simulink model "PTC_MBDS_StringToNumber_Sample"  (R2013a)
settings: Solver=FixedStepDiscrete  SolverMode=SingleTasking  StartTime=0.0  StopTime=100  FixedStep=0.02  RelTol=1e-3
libraries: PTC_MBDS_LIB x13, simulink_extras x1
CloseFcn:
  | rtwprivate ssgencode ModelCloseRequest MOD_Function6
Description:
  | Model of an MBDS Application
settings Model: CovPath=/Model  CovMetricSettings=dcmtrwa  CovHTMLOptions=-aTS=1 -bRG=1 -bTC=0 -hTR=0 -nFC=0 -scm=1 -bcm=1  covSaveCumulativeToWorkspaceVar=off  CovSaveSingleToWorkspaceVar=off  Creator=uid60719  LastModifiedBy=sundeep.tuteja
settings DataIOCC: LimitDataPoints=off  MaxDataPoints=100  SignalLoggingSaveFormat=ModelDataLogs  SaveOutput=off  SignalLogging=off  SaveTime=off
settings OptimizationCC: InlineParams=on  InlineInvariantSignals=on  ExpressionDepthLimit=2147483647  StateBitsets=on  DataBitsets=on  EfficientFloat2IntCast=on
settings DebuggingCC: ConsistencyChecking=error  SignalInfNanChecking=error  AlgebraicLoopMsg=error  ArtificialAlgebraicLoopMsg=error  SaveWithParameterizedLinksMsg=none  BlockPriorityViolationMsg=error  MinStepSizeMsg=error  SolverPrmCheckMsg=error  InheritedTsInSrcMsg=none  DiscreteInheritContinuousMsg=error  MultiTaskCondExecSysMsg=none  SingleTaskRateTransMsg=warning  TasksWithSamePriorityMsg=error  SigSpecEnsureSampleTimeMsg=error  CheckMatrixSingularityMsg=error  ParameterUnderflowMsg=error  UnnecessaryDatatypeConvMsg=warning  VectorMatrixConversionMsg=error  FcnCallInpInsideContextMsg=UseLocalSettings  SignalLabelMismatchMsg=warning  SFcnCompatibilityMsg=warning  UniqueDataStoreMsg=error  BusObjectLabelMismatch=error  RootOutportRequireBusObject=error  ModelReferenceIOMsg=warning  ModelReferenceVersionMismatchMessage=warning  ModelReferenceIOMismatchMessage=warning  ModelReferenceCSMismatchMessage=warning  UnknownTsInhSupMsg=error
settings HardwareCC: ProdIntDivRoundTo=Zero  ProdEndianess=BigEndian  ProdHWDeviceType=Specified  TargetHWDeviceType=32-bit Generic  ProdEqTarget=off
settings RTWCC: GenerateReport=on  ProcessScript=grt_make_rtw_hook  CustomInclude=dir c:\projects\siemensVDO\SV_MBDS\PLCLibrary\PLC\SVDO_Include\  LaunchReport=on  IncludeERTFirstTime=on
settings GRTTargetCC: CombineOutputUpdateFcns=off  GRTInterface=on

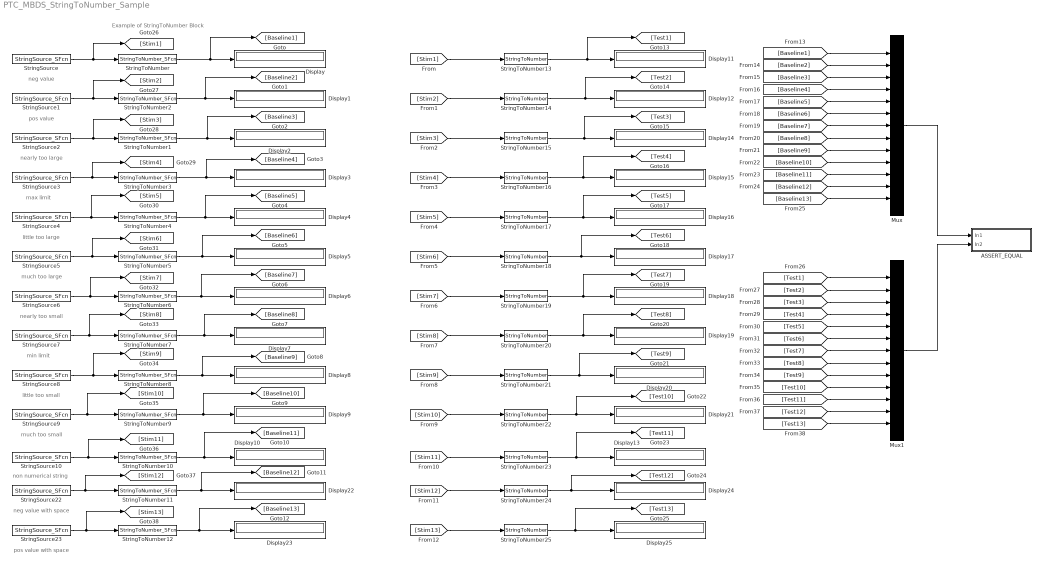
== system PTC_MBDS_StringToNumber_Sample ==
  note: neg value
  note: pos value
  note: nearly too large
  note: max limit
  note: little too large
  note: much too large
  note: nearly too small
  note: min limit
  note: little too small
  note: much too small
  note: non numerical string
  note: Example of StringToNumber Block
  note: neg value with space
  note: pos value with space
  ASSERT_EQUAL : Subsystem
  Display{,1..25} (26 alike) : Display
      settings: Format=decimal (Stored Integer)
  Mux : Mux  Inputs=13
  Mux1 : Mux  Inputs=13
  StringSource : S-Function  InitFcn=|  FunctionName=StringSource_SFcn  Parameters=uint8(String), uint16(MaxStringLength)  EnableBusSupport=off  mask(StringSource){MBDS_LibraryBlock=on, InputValue=-12345, MBDS_BlockVersion=05.20}
      | if(exist('MBDS_BlockCallback', 'file'))
      |    MBDS_BlockCallback('Update', gcb);
      | end
      mask prompts: MBDS_LibraryBlock "MBDS Library Block"; InputValue "Constant value:"; MBDS_BlockVersion "Block version:"
      mask help: This block outputs an uint8 array based on the ASCII codes of the string specified by the user.
      mask init:
      | MBDS_BlockCallback('Copy', gcb);
      | MaxStringLength = 1 + GetStringLen();
      | DispString = 'Error';
      | String = InputValue;
      | % Skip if string specifies a numeric expression or starts with '
      | if(isempty(str2num(String)) && String(1) ~= '''')
      |    try
      |       % Try to evaluate project constant 
      |       String = evalin('base', String);
      |    end   
      | end
      | if ~ischar(String) || size(String, 1) > 1
      | 	error('String must be a [1xn] array of type ''char'' with at least one character')
      | else
      |    % Limit to max. string length
      |    String = String(1:min(MaxStringLength, length(String)));
      | 	DispString = InputValue;
      | end
      mask Help: eval(['open([workdir(''Library_Dir:''),''\Blockset\Help\'',get_param(gcb,''MaskType''),''.html''])'])
      mask Display: text(0.05,0.5,DispString,'horizontalAlignment','left')
  StringSource1 : S-Function  InitFcn=|  FunctionName=StringSource_SFcn  Parameters=uint8(String), uint16(MaxStringLength)  EnableBusSupport=off  mask(StringSource){MBDS_LibraryBlock=on, InputValue=12345, MBDS_BlockVersion=05.20}
      | if(exist('MBDS_BlockCallback', 'file'))
      |    MBDS_BlockCallback('Update', gcb);
      | end
      mask prompts: MBDS_LibraryBlock "MBDS Library Block"; InputValue "Constant value:"; MBDS_BlockVersion "Block version:"
      mask help: This block outputs an uint8 array based on the ASCII codes of the string specified by the user.
      mask init: same as PTC_MBDS_StringToNumber_Sample/StringSource
      mask Help: eval(['open([workdir(''Library_Dir:''),''\Blockset\Help\'',get_param(gcb,''MaskType''),''.html''])'])
      mask Display: text(0.05,0.5,DispString,'horizontalAlignment','left')
  StringSource10 : S-Function  InitFcn=|  FunctionName=StringSource_SFcn  Parameters=uint8(String), uint16(MaxStringLength)  EnableBusSupport=off  mask(StringSource){MBDS_LibraryBlock=on, InputValue=1a23, MBDS_BlockVersion=05.20}
      | if(exist('MBDS_BlockCallback', 'file'))
      |    MBDS_BlockCallback('Update', gcb);
      | end
      mask prompts: MBDS_LibraryBlock "MBDS Library Block"; InputValue "Constant value:"; MBDS_BlockVersion "Block version:"
      mask help: This block outputs an uint8 array based on the ASCII codes of the string specified by the user.
      mask init: same as PTC_MBDS_StringToNumber_Sample/StringSource
      mask Help: eval(['open([workdir(''Library_Dir:''),''\Blockset\Help\'',get_param(gcb,''MaskType''),''.html''])'])
      mask Display: text(0.05,0.5,DispString,'horizontalAlignment','left')
  StringSource2 : S-Function  InitFcn=|  FunctionName=StringSource_SFcn  Parameters=uint8(String), uint16(MaxStringLength)  EnableBusSupport=off  mask(StringSource){MBDS_LibraryBlock=on, InputValue=2147483645, MBDS_BlockVersion=05.20}
      | if(exist('MBDS_BlockCallback', 'file'))
      |    MBDS_BlockCallback('Update', gcb);
      | end
      mask prompts: MBDS_LibraryBlock "MBDS Library Block"; InputValue "Constant value:"; MBDS_BlockVersion "Block version:"
      mask help: This block outputs an uint8 array based on the ASCII codes of the string specified by the user.
      mask init: same as PTC_MBDS_StringToNumber_Sample/StringSource
      mask Help: eval(['open([workdir(''Library_Dir:''),''\Blockset\Help\'',get_param(gcb,''MaskType''),''.html''])'])
      mask Display: text(0.05,0.5,DispString,'horizontalAlignment','left')
  StringSource22 : S-Function  InitFcn=|  FunctionName=StringSource_SFcn  Parameters=uint8(String), uint16(MaxStringLength)  EnableBusSupport=off  mask(StringSource){MBDS_LibraryBlock=on, InputValue=-12345, MBDS_BlockVersion=05.20}
      | if(exist('MBDS_BlockCallback', 'file'))
      |    MBDS_BlockCallback('Update', gcb);
      | end
      mask prompts: MBDS_LibraryBlock "MBDS Library Block"; InputValue "Constant value:"; MBDS_BlockVersion "Block version:"
      mask help: This block outputs an uint8 array based on the ASCII codes of the string specified by the user.
      mask init: same as PTC_MBDS_StringToNumber_Sample/StringSource
      mask Help: eval(['open([workdir(''Library_Dir:''),''\Blockset\Help\'',get_param(gcb,''MaskType''),''.html''])'])
      mask Display: text(0.05,0.5,DispString,'horizontalAlignment','left')
  StringSource23 : S-Function  InitFcn=|  FunctionName=StringSource_SFcn  Parameters=uint8(String), uint16(MaxStringLength)  EnableBusSupport=off  mask(StringSource){MBDS_LibraryBlock=on, InputValue=12345, MBDS_BlockVersion=05.20}
      | if(exist('MBDS_BlockCallback', 'file'))
      |    MBDS_BlockCallback('Update', gcb);
      | end
      mask prompts: MBDS_LibraryBlock "MBDS Library Block"; InputValue "Constant value:"; MBDS_BlockVersion "Block version:"
      mask help: This block outputs an uint8 array based on the ASCII codes of the string specified by the user.
      mask init: same as PTC_MBDS_StringToNumber_Sample/StringSource
      mask Help: eval(['open([workdir(''Library_Dir:''),''\Blockset\Help\'',get_param(gcb,''MaskType''),''.html''])'])
      mask Display: text(0.05,0.5,DispString,'horizontalAlignment','left')
  StringSource3 : S-Function  InitFcn=|  FunctionName=StringSource_SFcn  Parameters=uint8(String), uint16(MaxStringLength)  EnableBusSupport=off  mask(StringSource){MBDS_LibraryBlock=on, InputValue=2147483647, MBDS_BlockVersion=05.20}
      | if(exist('MBDS_BlockCallback', 'file'))
      |    MBDS_BlockCallback('Update', gcb);
      | end
      mask prompts: MBDS_LibraryBlock "MBDS Library Block"; InputValue "Constant value:"; MBDS_BlockVersion "Block version:"
      mask help: This block outputs an uint8 array based on the ASCII codes of the string specified by the user.
      mask init: same as PTC_MBDS_StringToNumber_Sample/StringSource
      mask Help: eval(['open([workdir(''Library_Dir:''),''\Blockset\Help\'',get_param(gcb,''MaskType''),''.html''])'])
      mask Display: text(0.05,0.5,DispString,'horizontalAlignment','left')
  StringSource4 : S-Function  InitFcn=|  FunctionName=StringSource_SFcn  Parameters=uint8(String), uint16(MaxStringLength)  EnableBusSupport=off  mask(StringSource){MBDS_LibraryBlock=on, InputValue=2147483648, MBDS_BlockVersion=05.20}
      | if(exist('MBDS_BlockCallback', 'file'))
      |    MBDS_BlockCallback('Update', gcb);
      | end
      mask prompts: MBDS_LibraryBlock "MBDS Library Block"; InputValue "Constant value:"; MBDS_BlockVersion "Block version:"
      mask help: This block outputs an uint8 array based on the ASCII codes of the string specified by the user.
      mask init: same as PTC_MBDS_StringToNumber_Sample/StringSource
      mask Help: eval(['open([workdir(''Library_Dir:''),''\Blockset\Help\'',get_param(gcb,''MaskType''),''.html''])'])
      mask Display: text(0.05,0.5,DispString,'horizontalAlignment','left')
  StringSource5 : S-Function  InitFcn=|  FunctionName=StringSource_SFcn  Parameters=uint8(String), uint16(MaxStringLength)  EnableBusSupport=off  mask(StringSource){MBDS_LibraryBlock=on, InputValue=12345678901, MBDS_BlockVersion=05.20}
      | if(exist('MBDS_BlockCallback', 'file'))
      |    MBDS_BlockCallback('Update', gcb);
      | end
      mask prompts: MBDS_LibraryBlock "MBDS Library Block"; InputValue "Constant value:"; MBDS_BlockVersion "Block version:"
      mask help: This block outputs an uint8 array based on the ASCII codes of the string specified by the user.
      mask init: same as PTC_MBDS_StringToNumber_Sample/StringSource
      mask Help: eval(['open([workdir(''Library_Dir:''),''\Blockset\Help\'',get_param(gcb,''MaskType''),''.html''])'])
      mask Display: text(0.05,0.5,DispString,'horizontalAlignment','left')
  StringSource6 : S-Function  InitFcn=|  FunctionName=StringSource_SFcn  Parameters=uint8(String), uint16(MaxStringLength)  EnableBusSupport=off  mask(StringSource){MBDS_LibraryBlock=on, InputValue=-2147483647, MBDS_BlockVersion=05.20}
      | if(exist('MBDS_BlockCallback', 'file'))
      |    MBDS_BlockCallback('Update', gcb);
      | end
      mask prompts: MBDS_LibraryBlock "MBDS Library Block"; InputValue "Constant value:"; MBDS_BlockVersion "Block version:"
      mask help: This block outputs an uint8 array based on the ASCII codes of the string specified by the user.
      mask init: same as PTC_MBDS_StringToNumber_Sample/StringSource
      mask Help: eval(['open([workdir(''Library_Dir:''),''\Blockset\Help\'',get_param(gcb,''MaskType''),''.html''])'])
      mask Display: text(0.05,0.5,DispString,'horizontalAlignment','left')
  StringSource7 : S-Function  InitFcn=|  FunctionName=StringSource_SFcn  Parameters=uint8(String), uint16(MaxStringLength)  EnableBusSupport=off  mask(StringSource){MBDS_LibraryBlock=on, InputValue=-2147483648, MBDS_BlockVersion=05.20}
      | if(exist('MBDS_BlockCallback', 'file'))
      |    MBDS_BlockCallback('Update', gcb);
      | end
      mask prompts: MBDS_LibraryBlock "MBDS Library Block"; InputValue "Constant value:"; MBDS_BlockVersion "Block version:"
      mask help: This block outputs an uint8 array based on the ASCII codes of the string specified by the user.
      mask init: same as PTC_MBDS_StringToNumber_Sample/StringSource
      mask Help: eval(['open([workdir(''Library_Dir:''),''\Blockset\Help\'',get_param(gcb,''MaskType''),''.html''])'])
      mask Display: text(0.05,0.5,DispString,'horizontalAlignment','left')
  StringSource8 : S-Function  InitFcn=|  FunctionName=StringSource_SFcn  Parameters=uint8(String), uint16(MaxStringLength)  EnableBusSupport=off  mask(StringSource){MBDS_LibraryBlock=on, InputValue=-2147483649, MBDS_BlockVersion=05.20}
      | if(exist('MBDS_BlockCallback', 'file'))
      |    MBDS_BlockCallback('Update', gcb);
      | end
      mask prompts: MBDS_LibraryBlock "MBDS Library Block"; InputValue "Constant value:"; MBDS_BlockVersion "Block version:"
      mask help: This block outputs an uint8 array based on the ASCII codes of the string specified by the user.
      mask init: same as PTC_MBDS_StringToNumber_Sample/StringSource
      mask Help: eval(['open([workdir(''Library_Dir:''),''\Blockset\Help\'',get_param(gcb,''MaskType''),''.html''])'])
      mask Display: text(0.05,0.5,DispString,'horizontalAlignment','left')
  StringSource9 : S-Function  InitFcn=|  FunctionName=StringSource_SFcn  Parameters=uint8(String), uint16(MaxStringLength)  EnableBusSupport=off  mask(StringSource){MBDS_LibraryBlock=on, InputValue=-12345678901, MBDS_BlockVersion=05.20}
      | if(exist('MBDS_BlockCallback', 'file'))
      |    MBDS_BlockCallback('Update', gcb);
      | end
      mask prompts: MBDS_LibraryBlock "MBDS Library Block"; InputValue "Constant value:"; MBDS_BlockVersion "Block version:"
      mask help: This block outputs an uint8 array based on the ASCII codes of the string specified by the user.
      mask init: same as PTC_MBDS_StringToNumber_Sample/StringSource
      mask Help: eval(['open([workdir(''Library_Dir:''),''\Blockset\Help\'',get_param(gcb,''MaskType''),''.html''])'])
      mask Display: text(0.05,0.5,DispString,'horizontalAlignment','left')
  StringToNumber : S-Function  InitFcn=|  FunctionName=StringToNumber_SFcn  Parameters=uint16(MaxStringLength)  EnableBusSupport=off  mask(StringToNumber){MBDS_LibraryBlock=on, MBDS_BlockVersion=05.40}
      | if(exist('MBDS_BlockCallback', 'file'))
      |    MBDS_BlockCallback('Update', gcb);
      | end
      mask prompts: MBDS_LibraryBlock "MBDS Library Block"; MBDS_BlockVersion "Block version:"
      mask help: Converts a numerical string to a number.
      mask init:
      | MBDS_BlockCallback('Copy', gcb);
      | MaxStringLength = 1 + GetStringLen();
      mask Help: eval(['open([workdir(''Library_Dir:''),''\Blockset\Help\'',get_param(gcb,''MaskType''),''.html''])'])
      mask Display: disp(['String -> Num'])
  StringToNumber1 : S-Function  InitFcn=|  FunctionName=StringToNumber_SFcn  Parameters=uint16(MaxStringLength)  EnableBusSupport=off  mask(StringToNumber){MBDS_LibraryBlock=on, MBDS_BlockVersion=05.40}
      | if(exist('MBDS_BlockCallback', 'file'))
      |    MBDS_BlockCallback('Update', gcb);
      | end
      mask prompts: MBDS_LibraryBlock "MBDS Library Block"; MBDS_BlockVersion "Block version:"
      mask help: Converts a numerical string to a number.
      mask init:
      | MBDS_BlockCallback('Copy', gcb);
      | MaxStringLength = 1 + GetStringLen();
      mask Help: eval(['open([workdir(''Library_Dir:''),''\Blockset\Help\'',get_param(gcb,''MaskType''),''.html''])'])
      mask Display: disp(['String -> Num'])
  StringToNumber10 : S-Function  InitFcn=|  FunctionName=StringToNumber_SFcn  Parameters=uint16(MaxStringLength)  EnableBusSupport=off  mask(StringToNumber){MBDS_LibraryBlock=on, MBDS_BlockVersion=05.40}
      | if(exist('MBDS_BlockCallback', 'file'))
      |    MBDS_BlockCallback('Update', gcb);
      | end
      mask prompts: MBDS_LibraryBlock "MBDS Library Block"; MBDS_BlockVersion "Block version:"
      mask help: Converts a numerical string to a number.
      mask init:
      | MBDS_BlockCallback('Copy', gcb);
      | MaxStringLength = 1 + GetStringLen();
      mask Help: eval(['open([workdir(''Library_Dir:''),''\Blockset\Help\'',get_param(gcb,''MaskType''),''.html''])'])
      mask Display: disp(['String -> Num'])
  StringToNumber11 : S-Function  InitFcn=|  FunctionName=StringToNumber_SFcn  Parameters=uint16(MaxStringLength)  EnableBusSupport=off  mask(StringToNumber){MBDS_LibraryBlock=on, MBDS_BlockVersion=05.40}
      | if(exist('MBDS_BlockCallback', 'file'))
      |    MBDS_BlockCallback('Update', gcb);
      | end
      mask prompts: MBDS_LibraryBlock "MBDS Library Block"; MBDS_BlockVersion "Block version:"
      mask help: Converts a numerical string to a number.
      mask init:
      | MBDS_BlockCallback('Copy', gcb);
      | MaxStringLength = 1 + GetStringLen();
      mask Help: eval(['open([workdir(''Library_Dir:''),''\Blockset\Help\'',get_param(gcb,''MaskType''),''.html''])'])
      mask Display: disp(['String -> Num'])
  StringToNumber12 : S-Function  InitFcn=|  FunctionName=StringToNumber_SFcn  Parameters=uint16(MaxStringLength)  EnableBusSupport=off  mask(StringToNumber){MBDS_LibraryBlock=on, MBDS_BlockVersion=05.40}
      | if(exist('MBDS_BlockCallback', 'file'))
      |    MBDS_BlockCallback('Update', gcb);
      | end
      mask prompts: MBDS_LibraryBlock "MBDS Library Block"; MBDS_BlockVersion "Block version:"
      mask help: Converts a numerical string to a number.
      mask init:
      | MBDS_BlockCallback('Copy', gcb);
      | MaxStringLength = 1 + GetStringLen();
      mask Help: eval(['open([workdir(''Library_Dir:''),''\Blockset\Help\'',get_param(gcb,''MaskType''),''.html''])'])
      mask Display: disp(['String -> Num'])
  StringToNumber{13..25} (13 alike) : PTC_MBDS_LIB/MBDS Standard Library/Extended Operations/String Operations/StringToNumber  PTC_MBDS_BlockVersion=5.32  PTC_BlockType=PTC_MBDS_StringToNumber  MaxStringLength=PTC_MBDS_MaxStringLength_Fcn
  StringToNumber2 : S-Function  InitFcn=|  FunctionName=StringToNumber_SFcn  Parameters=uint16(MaxStringLength)  EnableBusSupport=off  mask(StringToNumber){MBDS_LibraryBlock=on, MBDS_BlockVersion=05.40}
      | if(exist('MBDS_BlockCallback', 'file'))
      |    MBDS_BlockCallback('Update', gcb);
      | end
      mask prompts: MBDS_LibraryBlock "MBDS Library Block"; MBDS_BlockVersion "Block version:"
      mask help: Converts a numerical string to a number.
      mask init:
      | MBDS_BlockCallback('Copy', gcb);
      | MaxStringLength = 1 + GetStringLen();
      mask Help: eval(['open([workdir(''Library_Dir:''),''\Blockset\Help\'',get_param(gcb,''MaskType''),''.html''])'])
      mask Display: disp(['String -> Num'])
  StringToNumber3 : S-Function  InitFcn=|  FunctionName=StringToNumber_SFcn  Parameters=uint16(MaxStringLength)  EnableBusSupport=off  mask(StringToNumber){MBDS_LibraryBlock=on, MBDS_BlockVersion=05.40}
      | if(exist('MBDS_BlockCallback', 'file'))
      |    MBDS_BlockCallback('Update', gcb);
      | end
      mask prompts: MBDS_LibraryBlock "MBDS Library Block"; MBDS_BlockVersion "Block version:"
      mask help: Converts a numerical string to a number.
      mask init:
      | MBDS_BlockCallback('Copy', gcb);
      | MaxStringLength = 1 + GetStringLen();
      mask Help: eval(['open([workdir(''Library_Dir:''),''\Blockset\Help\'',get_param(gcb,''MaskType''),''.html''])'])
      mask Display: disp(['String -> Num'])
  StringToNumber4 : S-Function  InitFcn=|  FunctionName=StringToNumber_SFcn  Parameters=uint16(MaxStringLength)  EnableBusSupport=off  mask(StringToNumber){MBDS_LibraryBlock=on, MBDS_BlockVersion=05.40}
      | if(exist('MBDS_BlockCallback', 'file'))
      |    MBDS_BlockCallback('Update', gcb);
      | end
      mask prompts: MBDS_LibraryBlock "MBDS Library Block"; MBDS_BlockVersion "Block version:"
      mask help: Converts a numerical string to a number.
      mask init:
      | MBDS_BlockCallback('Copy', gcb);
      | MaxStringLength = 1 + GetStringLen();
      mask Help: eval(['open([workdir(''Library_Dir:''),''\Blockset\Help\'',get_param(gcb,''MaskType''),''.html''])'])
      mask Display: disp(['String -> Num'])
  StringToNumber5 : S-Function  InitFcn=|  FunctionName=StringToNumber_SFcn  Parameters=uint16(MaxStringLength)  EnableBusSupport=off  mask(StringToNumber){MBDS_LibraryBlock=on, MBDS_BlockVersion=05.40}
      | if(exist('MBDS_BlockCallback', 'file'))
      |    MBDS_BlockCallback('Update', gcb);
      | end
      mask prompts: MBDS_LibraryBlock "MBDS Library Block"; MBDS_BlockVersion "Block version:"
      mask help: Converts a numerical string to a number.
      mask init:
      | MBDS_BlockCallback('Copy', gcb);
      | MaxStringLength = 1 + GetStringLen();
      mask Help: eval(['open([workdir(''Library_Dir:''),''\Blockset\Help\'',get_param(gcb,''MaskType''),''.html''])'])
      mask Display: disp(['String -> Num'])
  StringToNumber6 : S-Function  InitFcn=|  FunctionName=StringToNumber_SFcn  Parameters=uint16(MaxStringLength)  EnableBusSupport=off  mask(StringToNumber){MBDS_LibraryBlock=on, MBDS_BlockVersion=05.40}
      | if(exist('MBDS_BlockCallback', 'file'))
      |    MBDS_BlockCallback('Update', gcb);
      | end
      mask prompts: MBDS_LibraryBlock "MBDS Library Block"; MBDS_BlockVersion "Block version:"
      mask help: Converts a numerical string to a number.
      mask init:
      | MBDS_BlockCallback('Copy', gcb);
      | MaxStringLength = 1 + GetStringLen();
      mask Help: eval(['open([workdir(''Library_Dir:''),''\Blockset\Help\'',get_param(gcb,''MaskType''),''.html''])'])
      mask Display: disp(['String -> Num'])
  StringToNumber7 : S-Function  InitFcn=|  FunctionName=StringToNumber_SFcn  Parameters=uint16(MaxStringLength)  EnableBusSupport=off  mask(StringToNumber){MBDS_LibraryBlock=on, MBDS_BlockVersion=05.40}
      | if(exist('MBDS_BlockCallback', 'file'))
      |    MBDS_BlockCallback('Update', gcb);
      | end
      mask prompts: MBDS_LibraryBlock "MBDS Library Block"; MBDS_BlockVersion "Block version:"
      mask help: Converts a numerical string to a number.
      mask init:
      | MBDS_BlockCallback('Copy', gcb);
      | MaxStringLength = 1 + GetStringLen();
      mask Help: eval(['open([workdir(''Library_Dir:''),''\Blockset\Help\'',get_param(gcb,''MaskType''),''.html''])'])
      mask Display: disp(['String -> Num'])
  StringToNumber8 : S-Function  InitFcn=|  FunctionName=StringToNumber_SFcn  Parameters=uint16(MaxStringLength)  EnableBusSupport=off  mask(StringToNumber){MBDS_LibraryBlock=on, MBDS_BlockVersion=05.40}
      | if(exist('MBDS_BlockCallback', 'file'))
      |    MBDS_BlockCallback('Update', gcb);
      | end
      mask prompts: MBDS_LibraryBlock "MBDS Library Block"; MBDS_BlockVersion "Block version:"
      mask help: Converts a numerical string to a number.
      mask init:
      | MBDS_BlockCallback('Copy', gcb);
      | MaxStringLength = 1 + GetStringLen();
      mask Help: eval(['open([workdir(''Library_Dir:''),''\Blockset\Help\'',get_param(gcb,''MaskType''),''.html''])'])
      mask Display: disp(['String -> Num'])
  StringToNumber9 : S-Function  InitFcn=|  FunctionName=StringToNumber_SFcn  Parameters=uint16(MaxStringLength)  EnableBusSupport=off  mask(StringToNumber){MBDS_LibraryBlock=on, MBDS_BlockVersion=05.40}
      | if(exist('MBDS_BlockCallback', 'file'))
      |    MBDS_BlockCallback('Update', gcb);
      | end
      mask prompts: MBDS_LibraryBlock "MBDS Library Block"; MBDS_BlockVersion "Block version:"
      mask help: Converts a numerical string to a number.
      mask init:
      | MBDS_BlockCallback('Copy', gcb);
      | MaxStringLength = 1 + GetStringLen();
      mask Help: eval(['open([workdir(''Library_Dir:''),''\Blockset\Help\'',get_param(gcb,''MaskType''),''.html''])'])
      mask Display: disp(['String -> Num'])
  wires:
  StringToNumber8/1 -> [Baseline9], Display8/1
  StringSource8/1 -> StringToNumber8/1, [Stim9]
  StringToNumber/1 -> [Baseline1], Display/1
  StringToNumber2/1 -> [Baseline2], Display1/1
  StringSource1/1 -> StringToNumber2/1, [Stim2]
  StringToNumber5/1 -> [Baseline6], Display5/1
  StringSource5/1 -> StringToNumber5/1, [Stim6]
  StringToNumber1/1 -> [Baseline3], Display2/1
  StringSource2/1 -> StringToNumber1/1, [Stim3]
  StringSource3/1 -> StringToNumber3/1, [Stim4]
  StringSource4/1 -> StringToNumber4/1, [Stim5]
  StringToNumber6/1 -> [Baseline7], Display6/1
  StringSource6/1 -> StringToNumber6/1, [Stim7]
  StringToNumber7/1 -> [Baseline8], Display7/1
  StringSource7/1 -> StringToNumber7/1, [Stim8]
  StringToNumber9/1 -> [Baseline10], Display9/1
  StringSource9/1 -> StringToNumber9/1, [Stim10]
  StringToNumber4/1 -> [Baseline5], Display4/1
  StringToNumber3/1 -> [Baseline4], Display3/1
  StringSource10/1 -> StringToNumber10/1, [Stim11]
  StringToNumber10/1 -> [Baseline11], Display10/1
  StringSource/1 -> StringToNumber/1, [Stim1]
  StringToNumber21/1 -> [Test9], Display20/1
  [Stim9] -> StringToNumber21/1
  StringToNumber13/1 -> [Test1], Display11/1
  StringToNumber14/1 -> [Test2], Display12/1
  [Stim2] -> StringToNumber14/1
  StringToNumber18/1 -> [Test6], Display17/1
  [Stim6] -> StringToNumber18/1
  StringToNumber15/1 -> [Test3], Display14/1
  [Stim3] -> StringToNumber15/1
  [Stim4] -> StringToNumber16/1
  [Stim5] -> StringToNumber17/1
  StringToNumber19/1 -> [Test7], Display18/1
  [Stim7] -> StringToNumber19/1
  StringToNumber20/1 -> [Test8], Display19/1
  [Stim8] -> StringToNumber20/1
  StringToNumber22/1 -> [Test10], Display21/1
  [Stim10] -> StringToNumber22/1
  StringToNumber17/1 -> [Test5], Display16/1
  StringToNumber16/1 -> [Test4], Display15/1
  [Stim11] -> StringToNumber23/1
  StringToNumber23/1 -> [Test11], Display13/1
  [Stim1] -> StringToNumber13/1
  StringToNumber11/1 -> [Baseline12], Display22/1
  StringToNumber12/1 -> [Baseline13], Display23/1
  StringSource23/1 -> StringToNumber12/1, [Stim13]
  StringSource22/1 -> StringToNumber11/1, [Stim12]
  StringToNumber24/1 -> [Test12], Display24/1
  StringToNumber25/1 -> [Test13], Display25/1
  [Stim13] -> StringToNumber25/1
  [Stim12] -> StringToNumber24/1
  [Baseline5] -> Mux/5
  [Baseline4] -> Mux/4
  [Baseline6] -> Mux/6
  [Baseline3] -> Mux/3
  [Baseline7] -> Mux/7
  [Baseline2] -> Mux/2
  [Baseline8] -> Mux/8
  [Baseline1] -> Mux/1
  [Baseline9] -> Mux/9
  [Baseline10] -> Mux/10
  [Baseline11] -> Mux/11
  [Baseline12] -> Mux/12
  [Baseline13] -> Mux/13
  [Test4] -> Mux1/4
  [Test3] -> Mux1/3
  [Test10] -> Mux1/10
  [Test2] -> Mux1/2
  [Test13] -> Mux1/13
  [Test11] -> Mux1/11
  [Test9] -> Mux1/9
  [Test7] -> Mux1/7
  [Test6] -> Mux1/6
  [Test5] -> Mux1/5
  [Test12] -> Mux1/12
  [Test1] -> Mux1/1
  [Test8] -> Mux1/8
  Mux1/1 -> ASSERT_EQUAL/2(In2)
  Mux/1 -> ASSERT_EQUAL/1(In1)

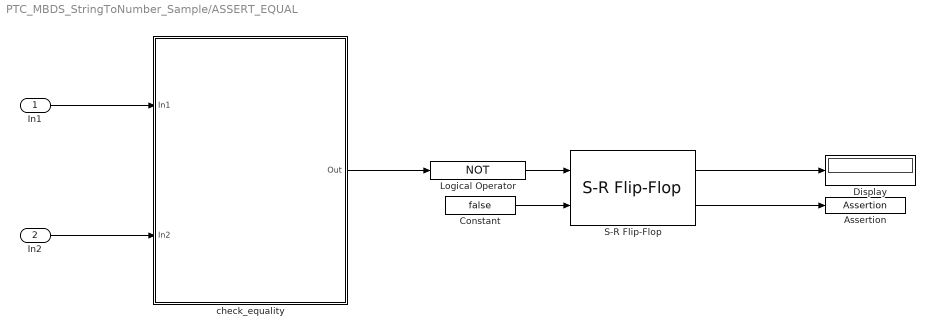
== system PTC_MBDS_StringToNumber_Sample/ASSERT_EQUAL ==
  In1 : Inport
  In2 : Inport  Port=2
  Assertion : Assertion
  Constant : Constant  Value=false
  Display : Display
  Logical Operator : Logic  Operator=NOT  AllPortsSameDT=off  OutDataTypeStr=boolean
  S-R Flip-Flop : simulink_extras/Flip Flops/S-R Flip-Flop  initial_condition=0
  check_equality : MATLAB Function  TreatAsAtomicUnit=on
  wires:
  S-R Flip-Flop/1 -> Display/1
  check_equality/1(Out) -> Logical Operator/1
  Constant/1 -> S-R Flip-Flop/2
  S-R Flip-Flop/2 -> Assertion/1
  In2/1 -> check_equality/2(In2)
  In1/1 -> check_equality/1(In1)
  Logical Operator/1 -> S-R Flip-Flop/1

== matlab function PTC_MBDS_StringToNumber_Sample/ASSERT_EQUAL/check_equality ==
  data: In1 input; Out output; In2 input
function Out = check_equality(In1, In2)
%#codegen

Out = isequaln(In1, In2);

end
